simulink model "Cruise_Control_Model"  (R2020a)
settings: Solver=ode45  StartTime=0.0  StopTime=15  RelTol=1e-3
values from neighbouring files (symbols this model uses):
  Af = 18    [Cruise_Control_Model.m]
  Cd = 0.3    [Cruise_Control_Model.m]
  gA = 4    [Cruise_Control_Model.m]
  Ka = 10    [Cruise_Control_Model.m]
  M = Wv/g    (= 96.3630711843)    [Cruise_Control_Model.m]
  rho = 0.0024    [Cruise_Control_Model.m]
  rw = 1    [Cruise_Control_Model.m]
  theta = 0.05    [Cruise_Control_Model.m]
  Vc = 88    [Cruise_Control_Model.m]
libraries: simulink x1, simulink_extras x1
settings Model: Creator=User  LastModifiedBy=Jayesh Patil
settings OptimizationCC: LifeSpan=inf
settings DebuggingCC: SFExecutionAtInitializationDiag=none  ArithmeticOperatorsInVariantConditions=warning
settings HardwareCC: ProdBitPerSizeT=32  ProdBitPerPtrDiffT=32  ProdWordSize=32  ProdHWDeviceType=Specified
settings SFSimCC: CustomCodeUndefinedFunction=UseInterfaceOnly
settings CodeAppCC: StateflowObjectComments=on

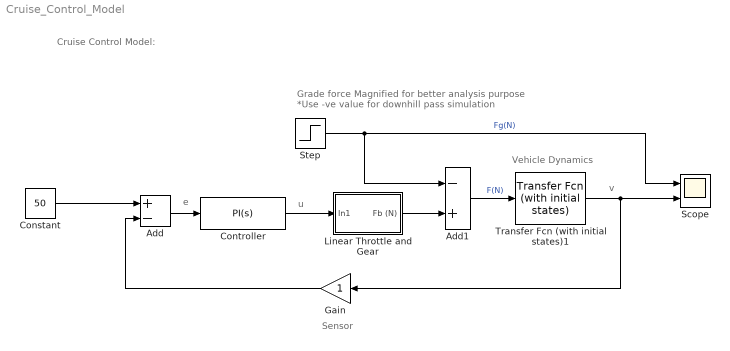
== system Cruise_Control_Model ==
  note: Grade force Magnified for better analysis purpose
      | *Use -ve value for downhill pass simulation
  note: v
  note: u
  note: e
  note: Cruise Control Model:
  note: Sensor
  note: Vehicle Dynamics
  Add : Sum  Inputs=+-
  Add1 : Sum  Inputs=-+
  Constant : Constant  Value=50
  Controller : simulink/Continuous/PID Controller  Controller=PI  Form=Parallel  TimeDomain=Continuous-time  UseExternalTs=off  SampleTime=-1  IntegratorMethod=Forward Euler  FilterMethod=Forward Euler  ControllerParametersSource=internal  P=10  I=50  D=0  UseFilter=on  N=100  TunerSelectOption=Transfer Function Based (PID Tuner App)  InitialConditionSource=internal  InitialConditionForIntegrator=0  InitialConditionForFilter=0  DifferentiatorICPrevScaledInput=0  ExternalReset=none  TrackingMode=off  Kt=1  LimitOutput=off  UpperSaturationLimit=inf  LowerSaturationLimit=-inf  LinearizeAsGain=on  AntiWindupMode=none  Kb=1  POutMin=[]  POutMax=[]  IOutMin=[]  IOutMax=[]  DOutMin=[]  DOutMax=[]  NOutMin=[]  NOutMax=[]  SumOutMin=[]  SumOutMax=[]  SaturationOutMin=[]  SaturationOutMax=[]  PParamMin=[]  PParamMax=[]  IParamMin=[]  IParamMax=[]  DParamMin=[]  DParamMax=[]  NParamMin=[]  NParamMax=[]  KbParamMin=[]  KbParamMax=[]  KtParamMin=[]  KtParamMax=[]  KbOutMin=[]  KbOutMax=[]  KtOutMin=[]  KtOutMax=[]  IntegratorOutMin=[]  IntegratorOutMax=[]  FilterOutMin=[]  FilterOutMax=[]  SumI1OutMin=[]  SumI1OutMax=[]  SumI2OutMin=[]  SumI2OutMax=[]  SumI3OutMin=[]  SumI3OutMax=[]  SumI4OutMin=[]  SumI4OutMax=[]  SumDOutMin=[]  SumDOutMax=[]  DifferentiatorOutMin=[]  DifferentiatorOutMax=[]  FilterDiffOutCoefMin=[]  FilterDiffOutCoefMax=[]  ReciprocalOutMin=[]  ReciprocalOutMax=[]  SumDenOutMin=[]  SumDenOutMax=[]  SumNumOutMin=[]  SumNumOutMax=[]  DivideOutMin=[]  DivideOutMax=[]  UdiffTsProdOutMin=[]  UdiffTsProdOutMax=[]  NTsProdOutMin=[]  NTsProdOutMax=[]  UintegralTsProdOutMin=[]  UintegralTsProdOutMax=[]  UngainTsProdOutMin=[]  UngainTsProdOutMax=[]  IntegratorContinuousStateAttributes=''  IntegratorStateMustResolveToSignalObject=off  IntegratorRTWStateStorageClass=Auto  FilterContinuousStateAttributes=''  FilterStateMustResolveToSignalObject=off  FilterRTWStateStorageClass=Auto  ParallelPVariant=InternalParameters  IdealPVariant=Disabled  IVariant=InternalParameters  DVariant=Disabled  IntegratorVariant=Continuous  SatVariant=Disabled  AWVariant=Passthrough  PCopyVariant=Disabled  TRVariant=Disabled  FdbkBlocksVariant=Forward  IdealPFdbkVariant=Disabled  SatFdbkVariant=Disabled  DerivativeFilterVariant=Disabled  NVariant=Disabled  NCopyVariant=Disabled_SignalSpec  FilterICVariant=Disabled  IntegratorICVariant=InternalICs  ExternalResetVariant=Disabled  TRSumVariant=Passthrough  SumFdbkVariant=Disabled  SumVariant=Sum_PI  TsampFilterVariant=InternalTs  TsampNgainVariant=Passthrough  TsampIntegralVariant=Passthrough  mask(PID 1dof){}
  Gain : Gain
  Linear Throttle and Gear : Subsystem
  Scope : Scope  NumInputPorts=2
  Step : Step  Time=5  After=M*theta*1000  SampleTime=0
  Transfer Fcn (with initial states)1 : simulink_extras/Additional Linear/Transfer Fcn (with initial states)  N=[1/M]  D="[1  rho*Cd*Af*Vc/M]"  X0=.5  mask(Transfer Function with Initial States){}
  wires:
  Add/1 -> Controller/1
  Gain/1 -> Add/2
  Constant/1 -> Add/1
  Step/1 -> Scope/1, Add1/1  "Fg(N)"
  Transfer Fcn (with initial states)1/1 -> Gain/1, Scope/2
  Add1/1 -> Transfer Fcn (with initial states)1/1  "F(N)"
  Controller/1 -> Linear Throttle and Gear/1(In1)
  Linear Throttle and Gear/1(Fb (N)) -> Add1/2

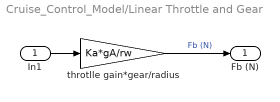
== system Cruise_Control_Model/Linear Throttle and Gear ==
  In1 : Inport
  throtlle gain*gear/radius : Gain  Gain=Ka*gA/rw
  Fb (N) : Outport
  wires:
  In1/1 -> throtlle gain*gear/radius/1
  throtlle gain*gear/radius/1 -> Fb (N)/1  "Fb (N)"
